simulink model "step2_compression_simulation"  (R2024b)
settings: Solver=VariableStepAuto  StartTime=0.0  StopTime=10  RelTol=1e-3
libraries: dspvision x1
settings Model: Creator=Egemen  LastModifiedBy=Egemen

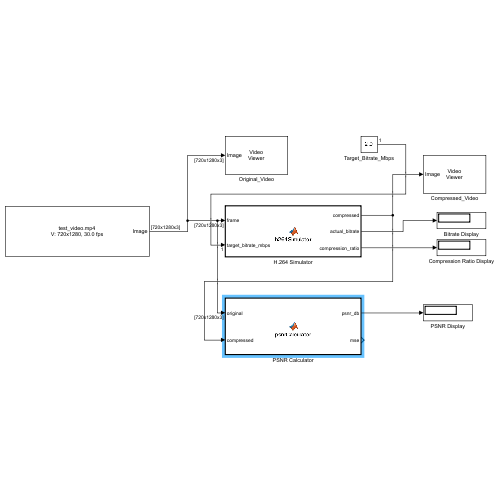
[thumbnail: Simulink's stored preview of the top-level diagram]
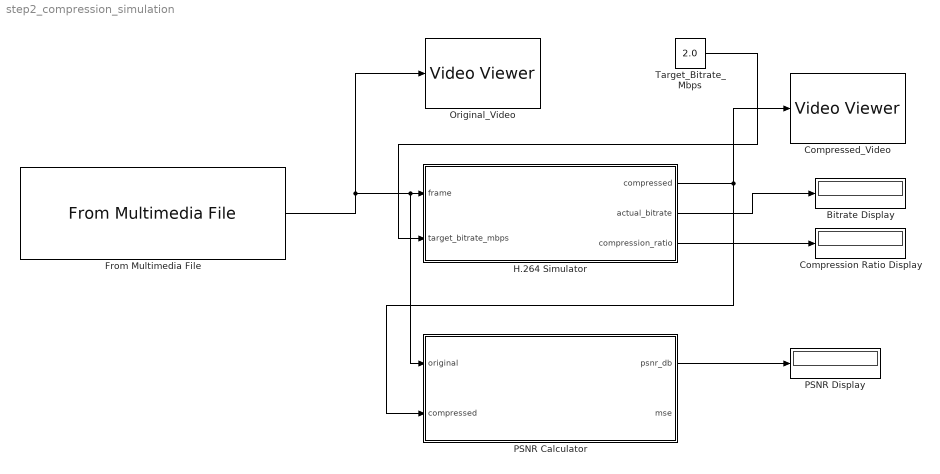
== system step2_compression_simulation ==
  Bitrate Display : Display
  Compressed_Video : VideoViewer  FigPos=[1 1038 1920 938]
  Compression Ratio Display : Display
  From Multimedia File : dspvision/From Multimedia File  inputFilename=C:\Users\Egemen\Documents\MATLAB\drone-video-bandwidth-optimization\scripts\initialization\data\input_videos\test_video.mp4  readRange=[1 Inf]  loop=on  numPlays=inf  outputStreams=Video only  videoDataType=single  audioDataType=int16  inheritSampleTime=off  userDefinedSampleTime=1/30  noAudioOutput=off  isIntensityVideo=off  fourcc=RGB  colorVideoFormat=One multidimensional signal  outputEOF=off  dataOrg=Column-major  audioFrameSize=1024  computeAudioFrameSize=off  outSamplingMode=Sample based
      settings: LibrarySourceBlock=visionsources/From Multimedia File
  H.264 Simulator : MATLAB Function  TreatAsAtomicUnit=on
  Original_Video : VideoViewer  FigPos=[1 1038 1920 938]
  PSNR Calculator : MATLAB Function  TreatAsAtomicUnit=on
  PSNR Display : Display
  Target_Bitrate_Mbps : Constant  Value=2.0  OutDataTypeStr=double
  wires:
  From Multimedia File/1 -> PSNR Calculator/1(original), H.264 Simulator/1(frame), Original_Video/1
  H.264 Simulator/1(compressed) -> PSNR Calculator/2(compressed), Compressed_Video/1
  PSNR Calculator/1(psnr_db) -> PSNR Display/1
  H.264 Simulator/2(actual_bitrate) -> Bitrate Display/1
  H.264 Simulator/3(compression_ratio) -> Compression Ratio Display/1
  Target_Bitrate_Mbps/1 -> H.264 Simulator/2(target_bitrate_mbps)

== matlab function step2_compression_simulation/PSNR Calculator ==
  data: original input; psnr_db output; compressed input; mse output
function [psnr_db, mse] = fcn(original, compressed)
    % PSNR Calculator - Minimal Version
    
    % Match sizes
    if ~isequal(size(original), size(compressed))
        compressed = imresize(compressed, [size(original,1), size(original,2)]);
    end
    
    % Convert to double
    o = double(original);
    c = double(compressed);
    
    % Calculate MSE
    mse = mean((o(:) - c(:)) .^ 2);
    
    % Calculate PSNR
    if mse < 1e-10
        psnr_db = 100.0;
    else
        psnr_db = 10.0 * log10(255.0 * 255.0 / mse);
    end
    
    % Clamp to valid range
    psnr_db = max(0.0, min(100.0, psnr_db));
end

== matlab function step2_compression_simulation/H.264 Simulator ==
  data: frame input; compressed output; target_bitrate_mbps input; actual_bitrate output; compression_ratio output
function [compressed, actual_bitrate, compression_ratio] = fcn(frame, target_bitrate_mbps)
    % H.264 Simulator - FINAL FIXED VERSION
    % Fixed size output, no dynamic allocation
    
    persistent frameCount totalBits;
    
    % Initialize persistent variables
    if isempty(frameCount)
        frameCount = uint32(0);
        totalBits = double(0);
    end
    
    % Get input dimensions
    inputSize = size(frame);
    
    % Validate input (must be 3D image)
    if length(inputSize) ~= 3 || inputSize(3) ~= 3
        % Return black frame with correct size
        compressed = uint8(zeros(720, 1280, 3));
        actual_bitrate = double(0);
        compression_ratio = double(1);
        return;
    end
    
    h = inputSize(1);
    w = inputSize(2);
    c = inputSize(3);
    
    % Check if frame is valid
    maxVal = double(max(frame(:)));
    if maxVal < 10
        % Too dark - return as is
        compressed = frame;
        actual_bitrate = double(0);
        compression_ratio = double(1);
        return;
    end
    
    % Increment counter
    frameCount = frameCount + uint32(1);
    
    %% COMPRESSION ALGORITHM
    
    % Calculate quality factor (0.2 to 1.0)
    quality = double(target_bitrate_mbps) / 8.0;
    if quality < 0.2
        quality = 0.2;
    end
    if quality > 1.0
        quality = 1.0;
    end
    
    % Scale factor for downsampling
    scaleFactor = 0.4 + 0.6 * quality;
    
    % PRE-ALLOCATE output with EXACT input size and UINT8 type
    compressed = uint8(zeros(h, w, c));
    
    % Process each color channel
    for channel = 1:c
        % Extract channel and convert to double for processing
        channelData = double(frame(:, :, channel));
        
        % Apply compression
        if scaleFactor < 0.99
            % Downsample
            smallImage = imresize(channelData, scaleFactor, 'bilinear');
            % Upsample back to original size
            processedData = imresize(smallImage, [h, w], 'bilinear');
        else
            processedData = channelData;
        end
        
        % Quantization (simulate information loss)
        if quality < 0.8
            quantizationStep = 1.0 + 8.0 * (1.0 - quality);
            processedData = round(processedData / quantizationStep) * quantizationStep;
        end
        
        % Add blur (compression artifacts)
        if quality < 0.7
            blurKernel = fspecial('average', 3);
            processedData = imfilter(processedData, blurKernel, 'replicate');
        end
        
        % Clamp values to valid range [0, 255]
        processedData(processedData < 0) = 0;
        processedData(processedData > 255) = 255;
        
        % Convert to uint8 and assign DIRECTLY
        compressed(:, :, channel) = uint8(round(processedData));
    end
    
    %% BITRATE CALCULATION
    
    % Original size in bits
    originalBits = double(h) * double(w) * double(c) * 8.0;
    
    % Compression efficiency (85% to 98% reduction)
    compressionEfficiency = 0.85 + 0.13 * quality;
    
    % Compressed size in bits
    compressedBits = originalBits * (1.0 - compressionEfficiency);
    
    % Accumulate total bits
    totalBits = totalBits + compressedBits;
    
    % Calculate average bitrate (Mbps)
    fps = 30.0;
    elapsedTime = double(frameCount) / fps;
    
    if elapsedTime > 0.001
        actual_bitrate = (totalBits / elapsedTime) / 1.0e6;
    else
        actual_bitrate = double(target_bitrate_mbps);
    end
    
    % Calculate compression ratio
    if compressedBits > 0.001
        compression_ratio = originalBits / compressedBits;
    else
        compression_ratio = double(1);
    end
end
